simulink model "Improved_version_succesful2"  (Simulink 7.3)
settings: Solver=ode45  StartTime=0.0  StopTime=.25  RelTol=1e-3
values from neighbouring files (symbols this model uses):
  y = 0.01    [objectivefcn.m]
undefined symbols (not defined in the file or in its folder): x
libraries: powerlib x176, powerlib_extras x120
(part 1 of 3)
settings Model: Creator=me  LastModifiedBy=me

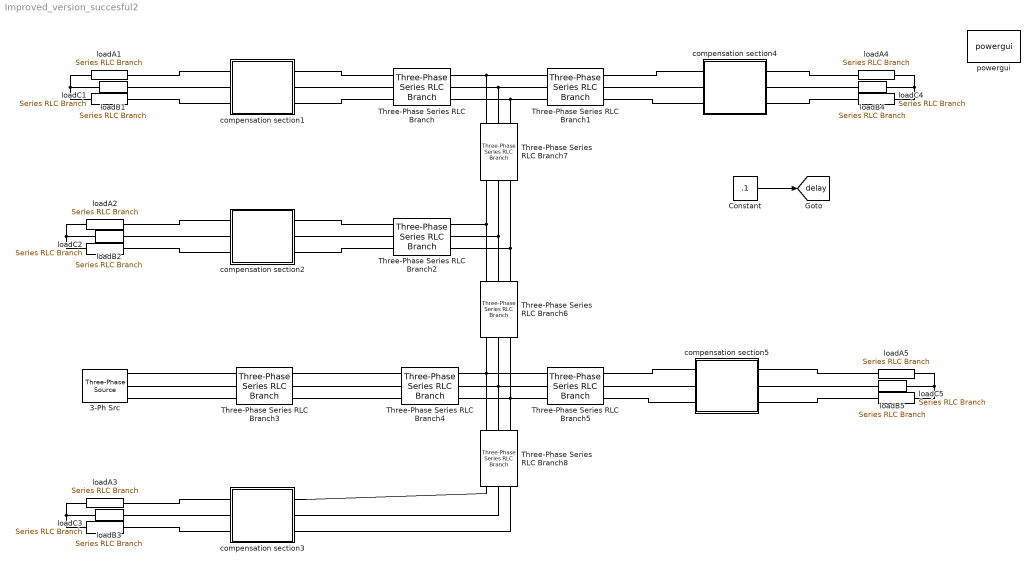
== system Improved_version_succesful2 ==
  3-Ph Src : powerlib/Electrical Sources/Three-Phase Source  DialogController=POWERSYS.PowerSysDialog  SystemSampleTime=-1  Voltage=380  PhaseAngle=0  Frequency=50  InternalConnection=Yn  SpecifyImpedance=on  Resistance=0.8929  Inductance=16.58e-3  ShortCircuitLevel=100e6  BaseVoltage=380  XRratio=7
  Constant : Constant  Value=.1  OutDataType=fixdt(1, 16)  OutScaling=2^0
  Three-Phase Series RLC Branch{,1..8} (9 alike) : powerlib/Elements/Three-Phase Series RLC Branch  DialogController=POWERSYS.PowerSysDialog  PhysicalDomain=powersysdomain  SubClassName=unknown  LeftPortType=p1  RightPortType=p1  LConnTagsString=A|B|C  RConnTagsString=A|B|C  BranchType=RL  Resistance=1  Inductance=1e-3  Capacitance=1e-6  Measurements=None
  compensation section1 : Subsystem
  compensation section2 : Subsystem
  compensation section3 : Subsystem
  compensation section4 : Subsystem
  compensation section5 : Subsystem
  loadA1 : powerlib/Elements/Series RLC Branch  DialogController=POWERSYS.PowerSysDialog  PhysicalDomain=powersysdomain  SubClassName=unknown  LeftPortType=p1  RightPortType=p1  LConnTagsString=__new0  RConnTagsString=__new0  BranchType=Open circuit  Resistance=10  Inductance=30/(100*pi)  SetiL0=off  InitialCurrent=0  Capacitance=1/(100*pi)  Setx0=off  InitialVoltage=0  Measurements=None
  loadA2 : powerlib/Elements/Series RLC Branch  DialogController=POWERSYS.PowerSysDialog  PhysicalDomain=powersysdomain  SubClassName=unknown  LeftPortType=p1  RightPortType=p1  LConnTagsString=__new0  RConnTagsString=__new0  BranchType=RL  Resistance=25  Inductance=30/(100*pi)  SetiL0=off  InitialCurrent=0  Capacitance=1/(100*pi)  Setx0=off  InitialVoltage=0  Measurements=None
  loadA3 : powerlib/Elements/Series RLC Branch  DialogController=POWERSYS.PowerSysDialog  PhysicalDomain=powersysdomain  SubClassName=unknown  LeftPortType=p1  RightPortType=p1  LConnTagsString=__new0  RConnTagsString=__new0  BranchType=R  Resistance=42  Inductance=30/(100*pi)  SetiL0=off  InitialCurrent=0  Capacitance=1/(100*pi)  Setx0=off  InitialVoltage=0  Measurements=None
  loadA4 : powerlib/Elements/Series RLC Branch  DialogController=POWERSYS.PowerSysDialog  PhysicalDomain=powersysdomain  SubClassName=unknown  LeftPortType=p1  RightPortType=p1  LConnTagsString=__new0  RConnTagsString=__new0  BranchType=RL  Resistance=10  Inductance=3/(100*pi)  SetiL0=off  InitialCurrent=0  Capacitance=1/(100*pi)  Setx0=off  InitialVoltage=0  Measurements=None
  loadA5 : powerlib/Elements/Series RLC Branch  DialogController=POWERSYS.PowerSysDialog  PhysicalDomain=powersysdomain  SubClassName=unknown  LeftPortType=p1  RightPortType=p1  LConnTagsString=__new0  RConnTagsString=__new0  BranchType=RL  Resistance=27  Inductance=35/(100*pi)  SetiL0=off  InitialCurrent=0  Capacitance=1/(100*pi)  Setx0=off  InitialVoltage=0  Measurements=None
  loadB1 : powerlib/Elements/Series RLC Branch  DialogController=POWERSYS.PowerSysDialog  PhysicalDomain=powersysdomain  SubClassName=unknown  LeftPortType=p1  RightPortType=p1  LConnTagsString=__new0  RConnTagsString=__new0  BranchType=RC  Resistance=23  Inductance=50/(100*pi)  SetiL0=off  InitialCurrent=0  Capacitance=1/(1200*pi)  Setx0=off  InitialVoltage=0  Measurements=None
  loadB2 : powerlib/Elements/Series RLC Branch  DialogController=POWERSYS.PowerSysDialog  PhysicalDomain=powersysdomain  SubClassName=unknown  LeftPortType=p1  RightPortType=p1  LConnTagsString=__new0  RConnTagsString=__new0  BranchType=R  Resistance=31  Inductance=50/(100*pi)  SetiL0=off  InitialCurrent=0  Capacitance=1/(1200*pi)  Setx0=off  InitialVoltage=0  Measurements=None
  loadB3 : powerlib/Elements/Series RLC Branch  DialogController=POWERSYS.PowerSysDialog  PhysicalDomain=powersysdomain  SubClassName=unknown  LeftPortType=p1  RightPortType=p1  LConnTagsString=__new0  RConnTagsString=__new0  BranchType=C  Resistance=23  Inductance=50/(100*pi)  SetiL0=off  InitialCurrent=0  Capacitance=1/(1200*pi)  Setx0=off  InitialVoltage=0  Measurements=None
  loadB4 : powerlib/Elements/Series RLC Branch  DialogController=POWERSYS.PowerSysDialog  PhysicalDomain=powersysdomain  SubClassName=unknown  LeftPortType=p1  RightPortType=p1  LConnTagsString=__new0  RConnTagsString=__new0  BranchType=LC  Resistance=23  Inductance=12/(100*pi)  SetiL0=off  InitialCurrent=0  Capacitance=1/(2300*pi)  Setx0=off  InitialVoltage=0  Measurements=None
  loadB5 : powerlib/Elements/Series RLC Branch  DialogController=POWERSYS.PowerSysDialog  PhysicalDomain=powersysdomain  SubClassName=unknown  LeftPortType=p1  RightPortType=p1  LConnTagsString=__new0  RConnTagsString=__new0  BranchType=Open circuit  Resistance=23  Inductance=50/(100*pi)  SetiL0=off  InitialCurrent=0  Capacitance=1/(1200*pi)  Setx0=off  InitialVoltage=0  Measurements=None
  loadC1 : powerlib/Elements/Series RLC Branch  DialogController=POWERSYS.PowerSysDialog  PhysicalDomain=powersysdomain  SubClassName=unknown  LeftPortType=p1  RightPortType=p1  LConnTagsString=__new0  RConnTagsString=__new0  BranchType=RL  Resistance=14  Inductance=29/(100*pi)  SetiL0=off  InitialCurrent=0  Capacitance=1.0  Setx0=off  InitialVoltage=0  Measurements=None
  loadC2 : powerlib/Elements/Series RLC Branch  DialogController=POWERSYS.PowerSysDialog  PhysicalDomain=powersysdomain  SubClassName=unknown  LeftPortType=p1  RightPortType=p1  LConnTagsString=__new0  RConnTagsString=__new0  BranchType=RC  Resistance=14  Inductance=29/(100*pi)  SetiL0=off  InitialCurrent=0  Capacitance=1/(1000*pi)  Setx0=off  InitialVoltage=0  Measurements=None
  loadC3 : powerlib/Elements/Series RLC Branch  DialogController=POWERSYS.PowerSysDialog  PhysicalDomain=powersysdomain  SubClassName=unknown  LeftPortType=p1  RightPortType=p1  LConnTagsString=__new0  RConnTagsString=__new0  BranchType=RL  Resistance=14  Inductance=38/(100*pi)  SetiL0=off  InitialCurrent=0  Capacitance=1.0  Setx0=off  InitialVoltage=0  Measurements=None
  loadC4 : powerlib/Elements/Series RLC Branch  DialogController=POWERSYS.PowerSysDialog  PhysicalDomain=powersysdomain  SubClassName=unknown  LeftPortType=p1  RightPortType=p1  LConnTagsString=__new0  RConnTagsString=__new0  BranchType=Open circuit  Resistance=14  Inductance=29/(100*pi)  SetiL0=off  InitialCurrent=0  Capacitance=1  Setx0=off  InitialVoltage=0  Measurements=None
  loadC5 : powerlib/Elements/Series RLC Branch  DialogController=POWERSYS.PowerSysDialog  PhysicalDomain=powersysdomain  SubClassName=unknown  LeftPortType=p1  RightPortType=p1  LConnTagsString=__new0  RConnTagsString=__new0  BranchType=RC  Resistance=24  Inductance=29/(100*pi)  SetiL0=off  InitialCurrent=0  Capacitance=1/(100*pi)  Setx0=off  InitialVoltage=0  Measurements=None
  powergui : powerlib/powergui  Priority=1  SystemSampleTime=-1  SimulationMode=Continuous  SampleTime=50e-6  frequency=60  SPID=off  DisableSnubberDevices=off  DisableRonSwitches=off  DisableVfSwitches=off  SwTol=0  Interpol=off  frequencyindice=50  echomessages=off  HookPort=off  DisplayEquations=off  FunctionMessages=off  EnableUseOfTLC=off  x0status=blocks  RestoreLinks=warning  Frange=[0:2:500]  Ylog=off  Xlog=on  ShowGrid=off  save=off  variable=ZData  ZoomFFT=on  StartTime=0.0  cycles=1  DisplayStyle=1  fundamental=60  FreqAxis=off  MaxFrequency=1000  frequencyindicesteady=1  RmsSteady=1  display=off  Ts=0  methode=off
  tag scope: delay=global
  wires:
  Constant/1 -> [delay]
  connections:
  loadA1/RConn1 -- loadC1/RConn1 -- loadB1/RConn1
  loadB2/RConn1 -- loadA2/RConn1 -- loadC2/RConn1
  loadB3/RConn1 -- loadA3/RConn1 -- loadC3/RConn1
  loadA4/LConn1 -- loadC4/LConn1 -- loadB4/LConn1
  loadB5/LConn1 -- loadA5/LConn1 -- loadC5/LConn1
  3-Ph Src/RConn3 -- Three-Phase Series RLC Branch3/LConn3
  3-Ph Src/RConn2 -- Three-Phase Series RLC Branch3/LConn2
  3-Ph Src/RConn1 -- Three-Phase Series RLC Branch3/LConn1
  Three-Phase Series RLC Branch3/RConn1 -- Three-Phase Series RLC Branch4/LConn1
  Three-Phase Series RLC Branch3/RConn2 -- Three-Phase Series RLC Branch4/LConn2
  Three-Phase Series RLC Branch3/RConn3 -- Three-Phase Series RLC Branch4/LConn3
  Three-Phase Series RLC Branch8/LConn1 -- Three-Phase Series RLC Branch4/RConn1 -- Three-Phase Series RLC Branch5/LConn1 -- Three-Phase Series RLC Branch6/RConn1
  Three-Phase Series RLC Branch8/LConn2 -- Three-Phase Series RLC Branch4/RConn2 -- Three-Phase Series RLC Branch5/LConn2 -- Three-Phase Series RLC Branch6/RConn2
  Three-Phase Series RLC Branch8/LConn3 -- Three-Phase Series RLC Branch4/RConn3 -- Three-Phase Series RLC Branch5/LConn3 -- Three-Phase Series RLC Branch6/RConn3
  Three-Phase Series RLC Branch7/RConn1 -- Three-Phase Series RLC Branch2/RConn1 -- Three-Phase Series RLC Branch6/LConn1
  Three-Phase Series RLC Branch7/RConn2 -- Three-Phase Series RLC Branch2/RConn2 -- Three-Phase Series RLC Branch6/LConn2
  Three-Phase Series RLC Branch7/RConn3 -- Three-Phase Series RLC Branch2/RConn3 -- Three-Phase Series RLC Branch6/LConn3
  Three-Phase Series RLC Branch7/LConn1 -- Three-Phase Series RLC Branch/RConn1 -- Three-Phase Series RLC Branch1/LConn1
  Three-Phase Series RLC Branch7/LConn2 -- Three-Phase Series RLC Branch/RConn2 -- Three-Phase Series RLC Branch1/LConn2
  Three-Phase Series RLC Branch7/LConn3 -- Three-Phase Series RLC Branch/RConn3 -- Three-Phase Series RLC Branch1/LConn3
  compensation section1/LConn1 -- Three-Phase Series RLC Branch/LConn1
  compensation section1/LConn2 -- Three-Phase Series RLC Branch/LConn2
  compensation section1/LConn3 -- Three-Phase Series RLC Branch/LConn3
  compensation section1/RConn1 -- loadA1/LConn1
  compensation section1/RConn2 -- loadB1/LConn1
  loadC1/LConn1 -- compensation section1/RConn3
  compensation section2/LConn2 -- Three-Phase Series RLC Branch2/LConn2
  compensation section2/LConn3 -- Three-Phase Series RLC Branch2/LConn3
  compensation section2/RConn1 -- loadA2/LConn1
  loadB2/LConn1 -- compensation section2/RConn2
  compensation section2/RConn3 -- loadC2/LConn1
  compensation section3/RConn1 -- loadA3/LConn1
  compensation section3/RConn2 -- loadB3/LConn1
  compensation section3/RConn3 -- loadC3/LConn1
  compensation section3/LConn1 -- Three-Phase Series RLC Branch8/RConn1
  Three-Phase Series RLC Branch8/RConn2 -- compensation section3/LConn2
  Three-Phase Series RLC Branch8/RConn3 -- compensation section3/LConn3
  Three-Phase Series RLC Branch2/LConn1 -- compensation section2/LConn1
  compensation section4/LConn1 -- Three-Phase Series RLC Branch1/RConn1
  compensation section4/LConn2 -- Three-Phase Series RLC Branch1/RConn2
  Three-Phase Series RLC Branch1/RConn3 -- compensation section4/LConn3
  compensation section4/RConn1 -- loadA4/RConn1
  compensation section4/RConn2 -- loadB4/RConn1
  compensation section4/RConn3 -- loadC4/RConn1
  compensation section5/LConn1 -- Three-Phase Series RLC Branch5/RConn1
  Three-Phase Series RLC Branch5/RConn2 -- compensation section5/LConn2
  Three-Phase Series RLC Branch5/RConn3 -- compensation section5/LConn3
  compensation section5/RConn1 -- loadA5/RConn1
  compensation section5/RConn2 -- loadB5/RConn1
  compensation section5/RConn3 -- loadC5/RConn1

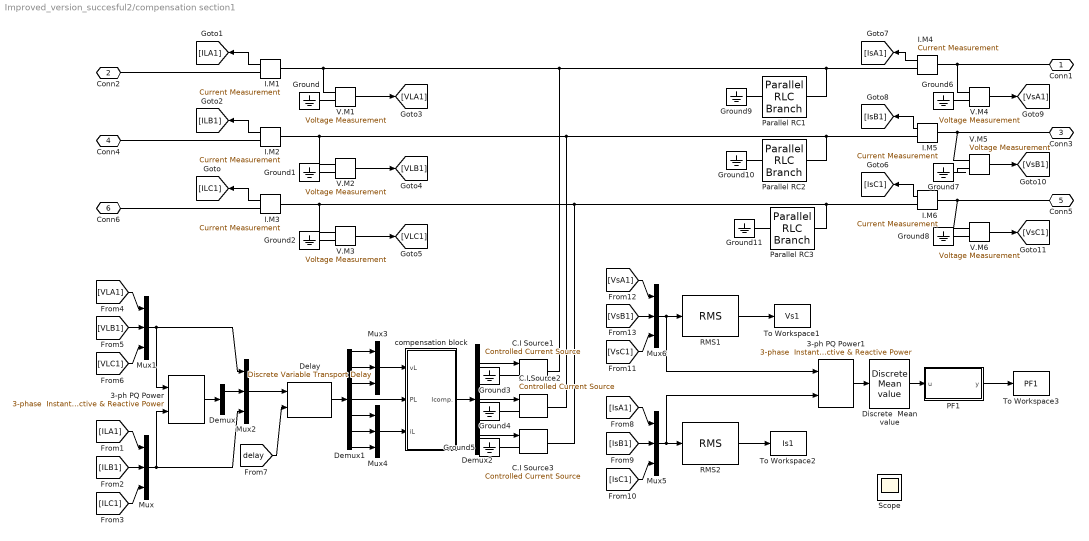
== system Improved_version_succesful2/compensation section1 ==
  3-ph PQ Power : powerlib_extras/Measurements/3-phase  Instantaneous  Active & Reactive Power  DialogController=POWERSYS.PowerSysDialog  SystemSampleTime=-1
  3-ph PQ Power1 : powerlib_extras/Measurements/3-phase  Instantaneous  Active & Reactive Power  DialogController=POWERSYS.PowerSysDialog  SystemSampleTime=-1
  C.I Source1 : powerlib/Electrical Sources/Controlled Current Source  DialogController=POWERSYS.PowerSysDialog  SystemSampleTime=-1  Initialize=on  Source_Type=AC  Amplitude=0  Phase=0  Frequency=0  Measurements=None
  C.I Source2 : powerlib/Electrical Sources/Controlled Current Source  DialogController=POWERSYS.PowerSysDialog  SystemSampleTime=-1  Initialize=on  Source_Type=AC  Amplitude=0  Phase=0  Frequency=0  Measurements=None
  C.I Source3 : powerlib/Electrical Sources/Controlled Current Source  DialogController=POWERSYS.PowerSysDialog  SystemSampleTime=-1  Initialize=on  Source_Type=AC  Amplitude=0  Phase=0  Frequency=0  Measurements=None
  Delay : powerlib_extras/Discrete  Control Blocks/Discrete Variable Transport Delay  DialogController=POWERSYS.PowerSysDialog  SystemSampleTime=-1  MaxDelay=1/40  InitialValue=0  Ts=50e-6
  Demux : Demux  Outputs=2
  Demux1 : Demux  Outputs=7
  Demux2 : Demux  Outputs=3
  Discrete  Mean value : powerlib_extras/Discrete Measurements/Discrete  Mean value  DialogController=POWERSYS.PowerSysDialog  SystemSampleTime=-1  Freq=50  Vinit=0  Ts=50e-6
  Ground{,1..11} (12 alike) : powerlib/Elements/Ground  DialogController=POWERSYS.PowerSysDialog  PhysicalDomain=powersysdomain  SubClassName=unknown  LeftPortType=p1  RightPortType=p1  LConnTagsString=a
  I.M{1..6} (6 alike) : powerlib/Measurements/Current Measurement  DialogController=POWERSYS.PowerSysDialog  SystemSampleTime=-1  PhasorSimulation=off  OutputType=Complex  PSBequivalent=0
  Mux{,1..6} (7 alike) : Mux  Inputs=3
  PF1 : Stateflow chart
  Parallel RC1 : powerlib/Elements/Parallel RLC Branch  DialogController=POWERSYS.PowerSysDialog  PhysicalDomain=powersysdomain  SubClassName=unknown  LeftPortType=p1  RightPortType=p1  LConnTagsString=a  RConnTagsString=__new0  BranchType=RC  Resistance=100  Inductance=1e-3  SetiL0=off  InitialCurrent=0  Capacitance=1/(10000*pi)  Setx0=off  InitialVoltage=0  Measurements=None
  Parallel RC2 : powerlib/Elements/Parallel RLC Branch  DialogController=POWERSYS.PowerSysDialog  PhysicalDomain=powersysdomain  SubClassName=unknown  LeftPortType=p1  RightPortType=p1  LConnTagsString=a  RConnTagsString=__new0  BranchType=RC  Resistance=100  Inductance=1e-3  SetiL0=off  InitialCurrent=0  Capacitance=1/(10000*pi)  Setx0=off  InitialVoltage=0  Measurements=None
  Parallel RC3 : powerlib/Elements/Parallel RLC Branch  DialogController=POWERSYS.PowerSysDialog  PhysicalDomain=powersysdomain  SubClassName=unknown  LeftPortType=p1  RightPortType=p1  LConnTagsString=a  RConnTagsString=__new0  BranchType=RC  Resistance=100  Inductance=1e-3  SetiL0=off  InitialCurrent=0  Capacitance=1/(10000*pi)  Setx0=off  InitialVoltage=0  Measurements=None
  RMS1 : powerlib_extras/Measurements/RMS  DialogController=POWERSYS.PowerSysDialog  SystemSampleTime=-1  f1=50
  RMS2 : powerlib_extras/Measurements/RMS  DialogController=POWERSYS.PowerSysDialog  SystemSampleTime=-1  f1=50
  Scope : Scope
      settings: YMin=2  YMax=6  SaveName=ScopeData2
  To Workspace1 : ToWorkspace  VariableName=Vs1  SampleTime=y  SaveFormat=Array
  To Workspace2 : ToWorkspace  VariableName=Is1  SampleTime=y  SaveFormat=Array
  To Workspace3 : ToWorkspace  VariableName=PF1  SampleTime=y  SaveFormat=Array
  V.M{1..6} (6 alike) : powerlib/Measurements/Voltage Measurement  DialogController=POWERSYS.PowerSysDialog  SystemSampleTime=-1  PhasorSimulation=off  OutputType=Complex  PSBequivalent=0
  compensation block : Subsystem
  Conn1 : PMIOPort  Port=1  Side=Left
  Conn2 : PMIOPort  Port=2  Side=Right
  Conn3 : PMIOPort  Port=3  Side=Left
  Conn4 : PMIOPort  Port=4  Side=Right
  Conn5 : PMIOPort  Port=5  Side=Left
  Conn6 : PMIOPort  Port=6  Side=Right
  wires:
  I.M1/1 -> [ILA1]
  I.M2/1 -> [ILB1]
  V.M1/1 -> [VLA1]
  V.M2/1 -> [VLB1]
  V.M3/1 -> [VLC1]
  [ILB1] -> Mux/2
  [ILA1] -> Mux/1
  [ILC1] -> Mux/3
  [VLB1] -> Mux1/2
  [VLA1] -> Mux1/1
  [VLC1] -> Mux1/3
  Mux1/1 -> Mux2/1, 3-ph PQ Power/1
  Mux/1 -> Mux2/3, 3-ph PQ Power/2
  3-ph PQ Power/1 -> Demux/1
  Demux/1 -> Mux2/2
  Mux2/1 -> Delay/1
  [delay] -> Delay/2
  Delay/1 -> Demux1/1
  Demux1/6 -> Mux4/2
  Demux1/5 -> Mux4/1
  Demux1/7 -> Mux4/3
  Demux1/1 -> Mux3/1
  Demux1/2 -> Mux3/2
  Demux1/3 -> Mux3/3
  Mux3/1 -> compensation block/1(vL)
  Demux1/4 -> compensation block/2(PL)
  Mux4/1 -> compensation block/3(iL)
  compensation block/1(Icomp.) -> Demux2/1
  Demux2/1 -> C.I Source1/1
  Demux2/2 -> C.I Source2/1
  Demux2/3 -> C.I Source3/1
  I.M3/1 -> [ILC1]
  I.M5/1 -> [IsB1]
  V.M4/1 -> [VsA1]
  V.M5/1 -> [VsB1]
  V.M6/1 -> [VsC1]
  I.M6/1 -> [IsC1]
  I.M4/1 -> [IsA1]
  [VsB1] -> Mux6/2
  [VsA1] -> Mux6/1
  [VsC1] -> Mux6/3
  Mux6/1 -> RMS1/1, 3-ph PQ Power1/1
  RMS1/1 -> To Workspace1/1
  [IsB1] -> Mux5/2
  [IsA1] -> Mux5/1
  [IsC1] -> Mux5/3
  Mux5/1 -> RMS2/1, 3-ph PQ Power1/2
  RMS2/1 -> To Workspace2/1
  3-ph PQ Power1/1 -> Discrete  Mean value/1
  Discrete  Mean value/1 -> PF1/1(u)
  PF1/1(y) -> To Workspace3/1
  connections:
  I.M1/LConn1 -- V.M1/LConn1 -- I.M4/RConn1 -- Parallel RC1/RConn1 -- C.I Source1/RConn1
  Conn2/RConn1 -- I.M1/RConn1
  I.M2/LConn1 -- V.M2/LConn1 -- I.M5/RConn1 -- Parallel RC2/RConn1 -- C.I Source2/RConn1
  Conn4/RConn1 -- I.M2/RConn1
  I.M3/LConn1 -- V.M3/LConn1 -- I.M6/RConn1 -- Parallel RC3/RConn1 -- C.I Source3/RConn1
  Ground/LConn1 -- V.M1/LConn2
  Ground1/LConn1 -- V.M2/LConn2
  Ground2/LConn1 -- V.M3/LConn2
  Ground5/LConn1 -- C.I Source3/LConn1
  Ground4/LConn1 -- C.I Source2/LConn1
  Ground3/LConn1 -- C.I Source1/LConn1
  Conn6/RConn1 -- I.M3/RConn1
  Conn1/RConn1 -- V.M4/LConn1 -- I.M4/LConn1
  V.M5/LConn1 -- I.M5/LConn1 -- Conn3/RConn1
  V.M6/LConn1 -- I.M6/LConn1 -- Conn5/RConn1
  Ground6/LConn1 -- V.M4/LConn2
  Ground7/LConn1 -- V.M5/LConn2
  Ground8/LConn1 -- V.M6/LConn2
  Parallel RC3/LConn1 -- Ground11/LConn1
  Parallel RC2/LConn1 -- Ground10/LConn1
  Parallel RC1/LConn1 -- Ground9/LConn1

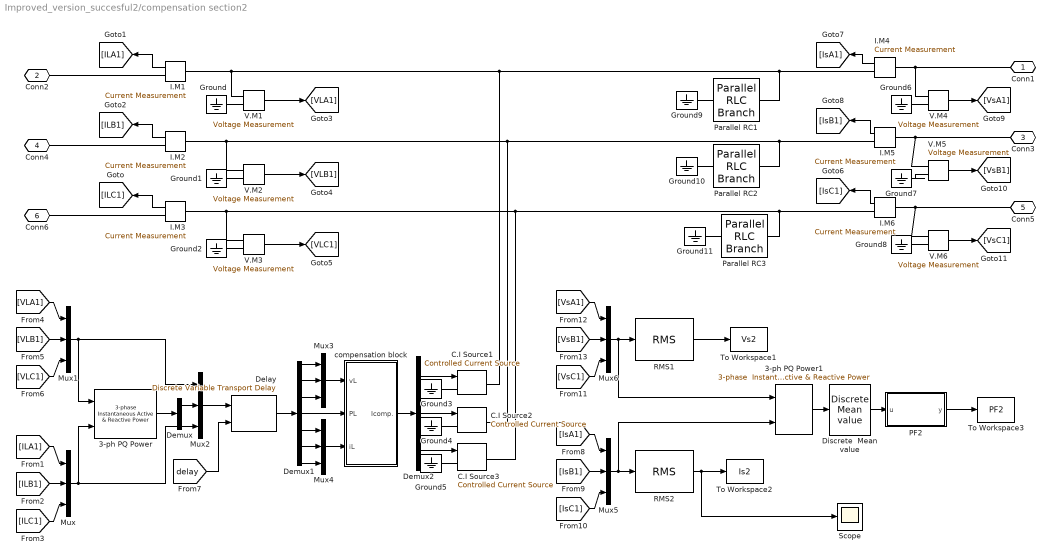
== system Improved_version_succesful2/compensation section2 ==
  3-ph PQ Power : powerlib_extras/Measurements/3-phase  Instantaneous  Active & Reactive Power  DialogController=POWERSYS.PowerSysDialog  SystemSampleTime=-1
  3-ph PQ Power1 : powerlib_extras/Measurements/3-phase  Instantaneous  Active & Reactive Power  DialogController=POWERSYS.PowerSysDialog  SystemSampleTime=-1
  C.I Source1 : powerlib/Electrical Sources/Controlled Current Source  DialogController=POWERSYS.PowerSysDialog  SystemSampleTime=-1  Initialize=on  Source_Type=AC  Amplitude=0  Phase=0  Frequency=0  Measurements=None
  C.I Source2 : powerlib/Electrical Sources/Controlled Current Source  DialogController=POWERSYS.PowerSysDialog  SystemSampleTime=-1  Initialize=on  Source_Type=AC  Amplitude=0  Phase=0  Frequency=0  Measurements=None
  C.I Source3 : powerlib/Electrical Sources/Controlled Current Source  DialogController=POWERSYS.PowerSysDialog  SystemSampleTime=-1  Initialize=on  Source_Type=AC  Amplitude=0  Phase=0  Frequency=0  Measurements=None
  Delay : powerlib_extras/Discrete  Control Blocks/Discrete Variable Transport Delay  DialogController=POWERSYS.PowerSysDialog  SystemSampleTime=-1  MaxDelay=1/40  InitialValue=0  Ts=50e-6
  Demux : Demux  Outputs=2
  Demux1 : Demux  Outputs=7
  Demux2 : Demux  Outputs=3
  Discrete  Mean value : powerlib_extras/Discrete Measurements/Discrete  Mean value  DialogController=POWERSYS.PowerSysDialog  SystemSampleTime=-1  Freq=50  Vinit=0  Ts=50e-6
  Ground{,1..11} (12 alike) : powerlib/Elements/Ground  DialogController=POWERSYS.PowerSysDialog  PhysicalDomain=powersysdomain  SubClassName=unknown  LeftPortType=p1  RightPortType=p1  LConnTagsString=a
  I.M{1..6} (6 alike) : powerlib/Measurements/Current Measurement  DialogController=POWERSYS.PowerSysDialog  SystemSampleTime=-1  PhasorSimulation=off  OutputType=Complex  PSBequivalent=0
  Mux{,1..6} (7 alike) : Mux  Inputs=3
  PF2 : Stateflow chart
  Parallel RC1 : powerlib/Elements/Parallel RLC Branch  DialogController=POWERSYS.PowerSysDialog  PhysicalDomain=powersysdomain  SubClassName=unknown  LeftPortType=p1  RightPortType=p1  LConnTagsString=a  RConnTagsString=__new0  BranchType=RC  Resistance=100  Inductance=1e-3  SetiL0=off  InitialCurrent=0  Capacitance=1/(10000*pi)  Setx0=off  InitialVoltage=0  Measurements=None
  Parallel RC2 : powerlib/Elements/Parallel RLC Branch  DialogController=POWERSYS.PowerSysDialog  PhysicalDomain=powersysdomain  SubClassName=unknown  LeftPortType=p1  RightPortType=p1  LConnTagsString=a  RConnTagsString=__new0  BranchType=RC  Resistance=100  Inductance=1e-3  SetiL0=off  InitialCurrent=0  Capacitance=1/(10000*pi)  Setx0=off  InitialVoltage=0  Measurements=None
  Parallel RC3 : powerlib/Elements/Parallel RLC Branch  DialogController=POWERSYS.PowerSysDialog  PhysicalDomain=powersysdomain  SubClassName=unknown  LeftPortType=p1  RightPortType=p1  LConnTagsString=a  RConnTagsString=__new0  BranchType=RC  Resistance=100  Inductance=1e-3  SetiL0=off  InitialCurrent=0  Capacitance=1/(10000*pi)  Setx0=off  InitialVoltage=0  Measurements=None
  RMS1 : powerlib_extras/Measurements/RMS  DialogController=POWERSYS.PowerSysDialog  SystemSampleTime=-1  f1=50
  RMS2 : powerlib_extras/Measurements/RMS  DialogController=POWERSYS.PowerSysDialog  SystemSampleTime=-1  f1=50
  Scope : Scope
      settings: YMin=4  YMax=10  SaveName=ScopeData3
  To Workspace1 : ToWorkspace  VariableName=Vs2  SampleTime=y  SaveFormat=Array
  To Workspace2 : ToWorkspace  VariableName=Is2  SampleTime=y  SaveFormat=Array
  To Workspace3 : ToWorkspace  VariableName=PF2  SampleTime=y  SaveFormat=Array
  V.M{1..6} (6 alike) : powerlib/Measurements/Voltage Measurement  DialogController=POWERSYS.PowerSysDialog  SystemSampleTime=-1  PhasorSimulation=off  OutputType=Complex  PSBequivalent=0
  compensation block : Subsystem
  Conn1 : PMIOPort  Port=1  Side=Left
  Conn2 : PMIOPort  Port=2  Side=Right
  Conn3 : PMIOPort  Port=3  Side=Left
  Conn4 : PMIOPort  Port=4  Side=Right
  Conn5 : PMIOPort  Port=5  Side=Left
  Conn6 : PMIOPort  Port=6  Side=Right
  wires:
  I.M4/1 -> [IsA1]
  I.M6/1 -> [IsC1]
  V.M6/1 -> [VsC1]
  V.M5/1 -> [VsB1]
  V.M4/1 -> [VsA1]
  I.M5/1 -> [IsB1]
  I.M3/1 -> [ILC1]
  Demux2/3 -> C.I Source3/1
  Demux2/2 -> C.I Source2/1
  Demux2/1 -> C.I Source1/1
  compensation block/1(Icomp.) -> Demux2/1
  Mux4/1 -> compensation block/3(iL)
  Demux1/4 -> compensation block/2(PL)
  Mux3/1 -> compensation block/1(vL)
  Demux1/3 -> Mux3/3
  Demux1/2 -> Mux3/2
  Demux1/1 -> Mux3/1
  Demux1/7 -> Mux4/3
  Demux1/5 -> Mux4/1
  Demux1/6 -> Mux4/2
  Delay/1 -> Demux1/1
  [delay] -> Delay/2
  Mux2/1 -> Delay/1
  Demux/1 -> Mux2/2
  3-ph PQ Power/1 -> Demux/1
  Mux/1 -> Mux2/3, 3-ph PQ Power/2
  Mux1/1 -> Mux2/1, 3-ph PQ Power/1
  [VLC1] -> Mux1/3
  [VLA1] -> Mux1/1
  [VLB1] -> Mux1/2
  [ILC1] -> Mux/3
  [ILA1] -> Mux/1
  [ILB1] -> Mux/2
  V.M3/1 -> [VLC1]
  V.M2/1 -> [VLB1]
  V.M1/1 -> [VLA1]
  I.M2/1 -> [ILB1]
  I.M1/1 -> [ILA1]
  [VsB1] -> Mux6/2
  [VsA1] -> Mux6/1
  [VsC1] -> Mux6/3
  Mux6/1 -> RMS1/1, 3-ph PQ Power1/1
  RMS1/1 -> To Workspace1/1
  [IsB1] -> Mux5/2
  [IsA1] -> Mux5/1
  [IsC1] -> Mux5/3
  Mux5/1 -> RMS2/1, 3-ph PQ Power1/2
  RMS2/1 -> To Workspace2/1, Scope/1
  3-ph PQ Power1/1 -> Discrete  Mean value/1
  Discrete  Mean value/1 -> PF2/1(u)
  PF2/1(y) -> To Workspace3/1
  connections:
  Parallel RC1/LConn1 -- Ground9/LConn1
  Parallel RC2/LConn1 -- Ground10/LConn1
  Parallel RC3/LConn1 -- Ground11/LConn1
  Ground8/LConn1 -- V.M6/LConn2
  Ground7/LConn1 -- V.M5/LConn2
  Ground6/LConn1 -- V.M4/LConn2
  Conn5/RConn1 -- I.M6/LConn1 -- V.M6/LConn1
  Conn3/RConn1 -- I.M5/LConn1 -- V.M5/LConn1
  I.M4/LConn1 -- V.M4/LConn1 -- Conn1/RConn1
  Conn6/RConn1 -- I.M3/RConn1
  Ground3/LConn1 -- C.I Source1/LConn1
  Ground4/LConn1 -- C.I Source2/LConn1
  Ground5/LConn1 -- C.I Source3/LConn1
  Ground2/LConn1 -- V.M3/LConn2
  Ground1/LConn1 -- V.M2/LConn2
  Ground/LConn1 -- V.M1/LConn2
  V.M3/LConn1 -- I.M3/LConn1 -- Parallel RC3/RConn1 -- I.M6/RConn1 -- C.I Source3/RConn1
  Conn4/RConn1 -- I.M2/RConn1
  V.M2/LConn1 -- I.M2/LConn1 -- Parallel RC2/RConn1 -- I.M5/RConn1 -- C.I Source2/RConn1
  Conn2/RConn1 -- I.M1/RConn1
  V.M1/LConn1 -- I.M1/LConn1 -- Parallel RC1/RConn1 -- I.M4/RConn1 -- C.I Source1/RConn1

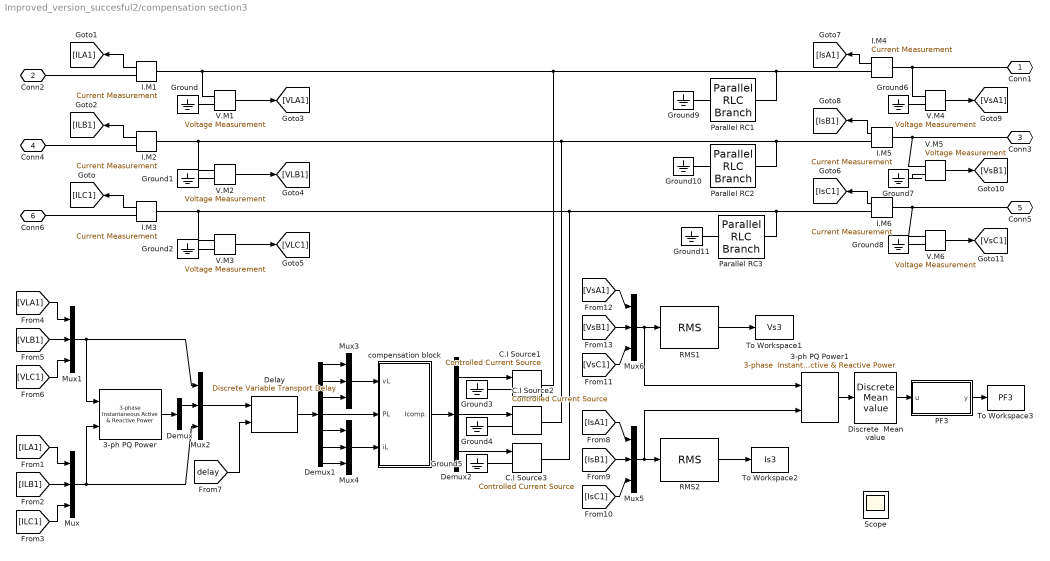
== system Improved_version_succesful2/compensation section3 ==
  3-ph PQ Power : powerlib_extras/Measurements/3-phase  Instantaneous  Active & Reactive Power  DialogController=POWERSYS.PowerSysDialog  SystemSampleTime=-1
  3-ph PQ Power1 : powerlib_extras/Measurements/3-phase  Instantaneous  Active & Reactive Power  DialogController=POWERSYS.PowerSysDialog  SystemSampleTime=-1
  C.I Source1 : powerlib/Electrical Sources/Controlled Current Source  DialogController=POWERSYS.PowerSysDialog  SystemSampleTime=-1  Initialize=on  Source_Type=AC  Amplitude=0  Phase=0  Frequency=0  Measurements=None
  C.I Source2 : powerlib/Electrical Sources/Controlled Current Source  DialogController=POWERSYS.PowerSysDialog  SystemSampleTime=-1  Initialize=on  Source_Type=AC  Amplitude=0  Phase=0  Frequency=0  Measurements=None
  C.I Source3 : powerlib/Electrical Sources/Controlled Current Source  DialogController=POWERSYS.PowerSysDialog  SystemSampleTime=-1  Initialize=on  Source_Type=AC  Amplitude=0  Phase=0  Frequency=0  Measurements=None
  Delay : powerlib_extras/Discrete  Control Blocks/Discrete Variable Transport Delay  DialogController=POWERSYS.PowerSysDialog  SystemSampleTime=-1  MaxDelay=1/40  InitialValue=0  Ts=50e-6
  Demux : Demux  Outputs=2
  Demux1 : Demux  Outputs=7
  Demux2 : Demux  Outputs=3
  Discrete  Mean value : powerlib_extras/Discrete Measurements/Discrete  Mean value  DialogController=POWERSYS.PowerSysDialog  SystemSampleTime=-1  Freq=50  Vinit=0  Ts=50e-6
  Ground{,1..11} (12 alike) : powerlib/Elements/Ground  DialogController=POWERSYS.PowerSysDialog  PhysicalDomain=powersysdomain  SubClassName=unknown  LeftPortType=p1  RightPortType=p1  LConnTagsString=a
  I.M{1..6} (6 alike) : powerlib/Measurements/Current Measurement  DialogController=POWERSYS.PowerSysDialog  SystemSampleTime=-1  PhasorSimulation=off  OutputType=Complex  PSBequivalent=0
  Mux{,1..6} (7 alike) : Mux  Inputs=3
  PF3 : Stateflow chart
  Parallel RC1 : powerlib/Elements/Parallel RLC Branch  DialogController=POWERSYS.PowerSysDialog  PhysicalDomain=powersysdomain  SubClassName=unknown  LeftPortType=p1  RightPortType=p1  LConnTagsString=a  RConnTagsString=__new0  BranchType=RC  Resistance=100  Inductance=1e-3  SetiL0=off  InitialCurrent=0  Capacitance=1/(10000*pi)  Setx0=off  InitialVoltage=0  Measurements=None
  Parallel RC2 : powerlib/Elements/Parallel RLC Branch  DialogController=POWERSYS.PowerSysDialog  PhysicalDomain=powersysdomain  SubClassName=unknown  LeftPortType=p1  RightPortType=p1  LConnTagsString=a  RConnTagsString=__new0  BranchType=RC  Resistance=100  Inductance=1e-3  SetiL0=off  InitialCurrent=0  Capacitance=1/(10000*pi)  Setx0=off  InitialVoltage=0  Measurements=None
  Parallel RC3 : powerlib/Elements/Parallel RLC Branch  DialogController=POWERSYS.PowerSysDialog  PhysicalDomain=powersysdomain  SubClassName=unknown  LeftPortType=p1  RightPortType=p1  LConnTagsString=a  RConnTagsString=__new0  BranchType=RC  Resistance=100  Inductance=1e-3  SetiL0=off  InitialCurrent=0  Capacitance=1/(10000*pi)  Setx0=off  InitialVoltage=0  Measurements=None
  RMS1 : powerlib_extras/Measurements/RMS  DialogController=POWERSYS.PowerSysDialog  SystemSampleTime=-1  f1=50
  RMS2 : powerlib_extras/Measurements/RMS  DialogController=POWERSYS.PowerSysDialog  SystemSampleTime=-1  f1=50
  Scope : Scope
      settings: YMin=2  YMax=6  SaveName=ScopeData4
  To Workspace1 : ToWorkspace  VariableName=Vs3  SampleTime=y  SaveFormat=Array
  To Workspace2 : ToWorkspace  VariableName=Is3  SampleTime=y  SaveFormat=Array
  To Workspace3 : ToWorkspace  VariableName=PF3  SampleTime=y  SaveFormat=Array
  V.M{1..6} (6 alike) : powerlib/Measurements/Voltage Measurement  DialogController=POWERSYS.PowerSysDialog  SystemSampleTime=-1  PhasorSimulation=off  OutputType=Complex  PSBequivalent=0
  compensation block : Subsystem
  Conn1 : PMIOPort  Port=1  Side=Left
  Conn2 : PMIOPort  Port=2  Side=Right
  Conn3 : PMIOPort  Port=3  Side=Left
  Conn4 : PMIOPort  Port=4  Side=Right
  Conn5 : PMIOPort  Port=5  Side=Left
  Conn6 : PMIOPort  Port=6  Side=Right
  wires:
  I.M1/1 -> [ILA1]
  I.M2/1 -> [ILB1]
  V.M1/1 -> [VLA1]
  V.M2/1 -> [VLB1]
  V.M3/1 -> [VLC1]
  [ILB1] -> Mux/2
  [ILA1] -> Mux/1
  [ILC1] -> Mux/3
  [VLB1] -> Mux1/2
  [VLA1] -> Mux1/1
  [VLC1] -> Mux1/3
  Mux1/1 -> 3-ph PQ Power/1, Mux2/1
  Mux/1 -> 3-ph PQ Power/2, Mux2/3
  3-ph PQ Power/1 -> Demux/1
  Demux/1 -> Mux2/2
  Mux2/1 -> Delay/1
  [delay] -> Delay/2
  Delay/1 -> Demux1/1
  Demux1/6 -> Mux4/2
  Demux1/5 -> Mux4/1
  Demux1/7 -> Mux4/3
  Demux1/1 -> Mux3/1
  Demux1/2 -> Mux3/2
  Demux1/3 -> Mux3/3
  Mux3/1 -> compensation block/1(vL)
  Demux1/4 -> compensation block/2(PL)
  Mux4/1 -> compensation block/3(iL)
  compensation block/1(Icomp.) -> Demux2/1
  Demux2/1 -> C.I Source1/1
  Demux2/2 -> C.I Source2/1
  Demux2/3 -> C.I Source3/1
  I.M3/1 -> [ILC1]
  I.M5/1 -> [IsB1]
  V.M4/1 -> [VsA1]
  V.M5/1 -> [VsB1]
  V.M6/1 -> [VsC1]
  I.M6/1 -> [IsC1]
  I.M4/1 -> [IsA1]
  [VsB1] -> Mux6/2
  [VsA1] -> Mux6/1
  [VsC1] -> Mux6/3
  Mux6/1 -> RMS1/1, 3-ph PQ Power1/1
  RMS1/1 -> To Workspace1/1
  [IsB1] -> Mux5/2
  [IsA1] -> Mux5/1
  [IsC1] -> Mux5/3
  Mux5/1 -> RMS2/1, 3-ph PQ Power1/2
  RMS2/1 -> To Workspace2/1
  3-ph PQ Power1/1 -> Discrete  Mean value/1
  Discrete  Mean value/1 -> PF3/1(u)
  PF3/1(y) -> To Workspace3/1
  connections:
  I.M1/LConn1 -- V.M1/LConn1 -- I.M4/RConn1 -- Parallel RC1/RConn1 -- C.I Source1/RConn1
  Conn2/RConn1 -- I.M1/RConn1
  I.M2/LConn1 -- V.M2/LConn1 -- I.M5/RConn1 -- Parallel RC2/RConn1 -- C.I Source2/RConn1
  Conn4/RConn1 -- I.M2/RConn1
  I.M3/LConn1 -- V.M3/LConn1 -- I.M6/RConn1 -- Parallel RC3/RConn1 -- C.I Source3/RConn1
  Ground/LConn1 -- V.M1/LConn2
  Ground1/LConn1 -- V.M2/LConn2
  Ground2/LConn1 -- V.M3/LConn2
  Ground5/LConn1 -- C.I Source3/LConn1
  Ground4/LConn1 -- C.I Source2/LConn1
  Ground3/LConn1 -- C.I Source1/LConn1
  Conn6/RConn1 -- I.M3/RConn1
  Conn1/RConn1 -- V.M4/LConn1 -- I.M4/LConn1
  V.M5/LConn1 -- I.M5/LConn1 -- Conn3/RConn1
  V.M6/LConn1 -- I.M6/LConn1 -- Conn5/RConn1
  Ground6/LConn1 -- V.M4/LConn2
  Ground7/LConn1 -- V.M5/LConn2
  Ground8/LConn1 -- V.M6/LConn2
  Parallel RC3/LConn1 -- Ground11/LConn1
  Parallel RC2/LConn1 -- Ground10/LConn1
  Parallel RC1/LConn1 -- Ground9/LConn1

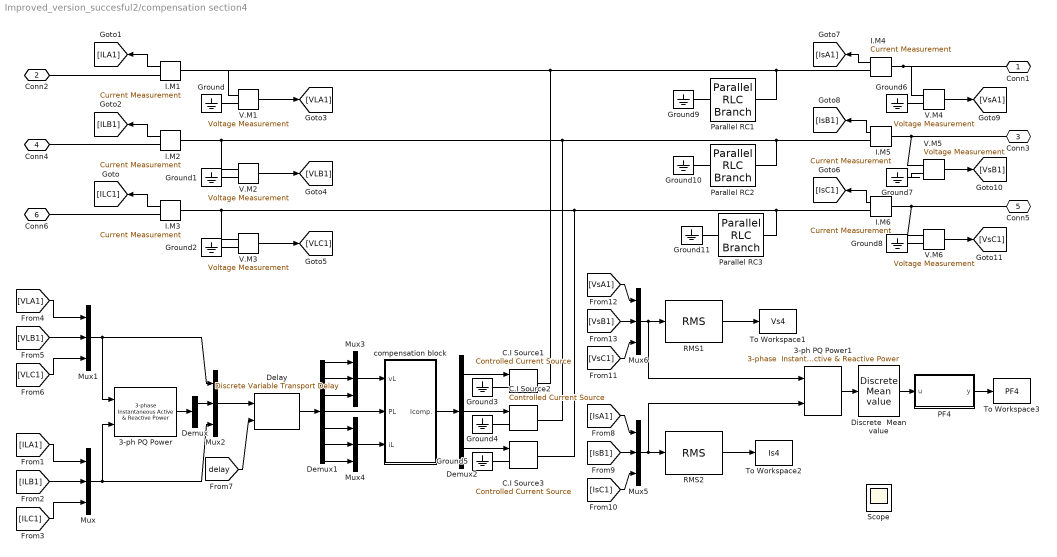
== system Improved_version_succesful2/compensation section4 ==
  3-ph PQ Power : powerlib_extras/Measurements/3-phase  Instantaneous  Active & Reactive Power  DialogController=POWERSYS.PowerSysDialog  SystemSampleTime=-1
  3-ph PQ Power1 : powerlib_extras/Measurements/3-phase  Instantaneous  Active & Reactive Power  DialogController=POWERSYS.PowerSysDialog  SystemSampleTime=-1
  C.I Source1 : powerlib/Electrical Sources/Controlled Current Source  DialogController=POWERSYS.PowerSysDialog  SystemSampleTime=-1  Initialize=on  Source_Type=AC  Amplitude=0  Phase=0  Frequency=0  Measurements=None
  C.I Source2 : powerlib/Electrical Sources/Controlled Current Source  DialogController=POWERSYS.PowerSysDialog  SystemSampleTime=-1  Initialize=on  Source_Type=AC  Amplitude=0  Phase=0  Frequency=0  Measurements=None
  C.I Source3 : powerlib/Electrical Sources/Controlled Current Source  DialogController=POWERSYS.PowerSysDialog  SystemSampleTime=-1  Initialize=on  Source_Type=AC  Amplitude=0  Phase=0  Frequency=0  Measurements=None
  Delay : powerlib_extras/Discrete  Control Blocks/Discrete Variable Transport Delay  DialogController=POWERSYS.PowerSysDialog  SystemSampleTime=-1  MaxDelay=1/40  InitialValue=0  Ts=50e-6
  Demux : Demux  Outputs=2
  Demux1 : Demux  Outputs=7
  Demux2 : Demux  Outputs=3
  Discrete  Mean value : powerlib_extras/Discrete Measurements/Discrete  Mean value  DialogController=POWERSYS.PowerSysDialog  SystemSampleTime=-1  Freq=50  Vinit=0  Ts=50e-6
  Ground{,1..11} (12 alike) : powerlib/Elements/Ground  DialogController=POWERSYS.PowerSysDialog  PhysicalDomain=powersysdomain  SubClassName=unknown  LeftPortType=p1  RightPortType=p1  LConnTagsString=a
  I.M{1..6} (6 alike) : powerlib/Measurements/Current Measurement  DialogController=POWERSYS.PowerSysDialog  SystemSampleTime=-1  PhasorSimulation=off  OutputType=Complex  PSBequivalent=0
  Mux{,1..6} (7 alike) : Mux  Inputs=3
  PF4 : Stateflow chart
  Parallel RC1 : powerlib/Elements/Parallel RLC Branch  DialogController=POWERSYS.PowerSysDialog  PhysicalDomain=powersysdomain  SubClassName=unknown  LeftPortType=p1  RightPortType=p1  LConnTagsString=a  RConnTagsString=__new0  BranchType=RC  Resistance=100  Inductance=1e-3  SetiL0=off  InitialCurrent=0  Capacitance=1/(10000*pi)  Setx0=off  InitialVoltage=0  Measurements=None
  Parallel RC2 : powerlib/Elements/Parallel RLC Branch  DialogController=POWERSYS.PowerSysDialog  PhysicalDomain=powersysdomain  SubClassName=unknown  LeftPortType=p1  RightPortType=p1  LConnTagsString=a  RConnTagsString=__new0  BranchType=RC  Resistance=100  Inductance=1e-3  SetiL0=off  InitialCurrent=0  Capacitance=1/(10000*pi)  Setx0=off  InitialVoltage=0  Measurements=None
  Parallel RC3 : powerlib/Elements/Parallel RLC Branch  DialogController=POWERSYS.PowerSysDialog  PhysicalDomain=powersysdomain  SubClassName=unknown  LeftPortType=p1  RightPortType=p1  LConnTagsString=a  RConnTagsString=__new0  BranchType=RC  Resistance=100  Inductance=1e-3  SetiL0=off  InitialCurrent=0  Capacitance=1/(10000*pi)  Setx0=off  InitialVoltage=0  Measurements=None
  RMS1 : powerlib_extras/Measurements/RMS  DialogController=POWERSYS.PowerSysDialog  SystemSampleTime=-1  f1=50
  RMS2 : powerlib_extras/Measurements/RMS  DialogController=POWERSYS.PowerSysDialog  SystemSampleTime=-1  f1=50
  Scope : Scope
      settings: YMin=2  YMax=6  SaveName=ScopeData5
  To Workspace1 : ToWorkspace  VariableName=Vs4  SampleTime=y  SaveFormat=Array
  To Workspace2 : ToWorkspace  VariableName=Is4  SampleTime=y  SaveFormat=Array
  To Workspace3 : ToWorkspace  VariableName=PF4  SampleTime=y  SaveFormat=Array
  V.M{1..6} (6 alike) : powerlib/Measurements/Voltage Measurement  DialogController=POWERSYS.PowerSysDialog  SystemSampleTime=-1  PhasorSimulation=off  OutputType=Complex  PSBequivalent=0
  compensation block : Subsystem
  Conn1 : PMIOPort  Port=1  Side=Left
  Conn2 : PMIOPort  Port=2  Side=Right
  Conn3 : PMIOPort  Port=3  Side=Left
  Conn4 : PMIOPort  Port=4  Side=Right
  Conn5 : PMIOPort  Port=5  Side=Left
  Conn6 : PMIOPort  Port=6  Side=Right
  wires:
  I.M4/1 -> [IsA1]
  I.M6/1 -> [IsC1]
  V.M6/1 -> [VsC1]
  V.M5/1 -> [VsB1]
  V.M4/1 -> [VsA1]
  I.M5/1 -> [IsB1]
  I.M3/1 -> [ILC1]
  Demux2/3 -> C.I Source3/1
  Demux2/2 -> C.I Source2/1
  Demux2/1 -> C.I Source1/1
  compensation block/1(Icomp.) -> Demux2/1
  Mux4/1 -> compensation block/3(iL)
  Demux1/4 -> compensation block/2(PL)
  Mux3/1 -> compensation block/1(vL)
  Demux1/3 -> Mux3/3
  Demux1/2 -> Mux3/2
  Demux1/1 -> Mux3/1
  Demux1/7 -> Mux4/3
  Demux1/5 -> Mux4/1
  Demux1/6 -> Mux4/2
  Delay/1 -> Demux1/1
  [delay] -> Delay/2
  Mux2/1 -> Delay/1
  Demux/1 -> Mux2/2
  3-ph PQ Power/1 -> Demux/1
  Mux/1 -> Mux2/3, 3-ph PQ Power/2
  Mux1/1 -> Mux2/1, 3-ph PQ Power/1
  [VLC1] -> Mux1/3
  [VLA1] -> Mux1/1
  [VLB1] -> Mux1/2
  [ILC1] -> Mux/3
  [ILA1] -> Mux/1
  [ILB1] -> Mux/2
  V.M3/1 -> [VLC1]
  V.M2/1 -> [VLB1]
  V.M1/1 -> [VLA1]
  I.M2/1 -> [ILB1]
  I.M1/1 -> [ILA1]
  [VsB1] -> Mux6/2
  [VsA1] -> Mux6/1
  [VsC1] -> Mux6/3
  Mux6/1 -> RMS1/1, 3-ph PQ Power1/1
  RMS1/1 -> To Workspace1/1
  [IsB1] -> Mux5/2
  [IsA1] -> Mux5/1
  [IsC1] -> Mux5/3
  Mux5/1 -> RMS2/1, 3-ph PQ Power1/2
  RMS2/1 -> To Workspace2/1
  3-ph PQ Power1/1 -> Discrete  Mean value/1
  Discrete  Mean value/1 -> PF4/1(u)
  PF4/1(y) -> To Workspace3/1
  connections:
  Parallel RC1/LConn1 -- Ground9/LConn1
  Parallel RC2/LConn1 -- Ground10/LConn1
  Parallel RC3/LConn1 -- Ground11/LConn1
  Ground8/LConn1 -- V.M6/LConn2
  Ground7/LConn1 -- V.M5/LConn2
  Ground6/LConn1 -- V.M4/LConn2
  Conn5/RConn1 -- I.M6/LConn1 -- V.M6/LConn1
  Conn3/RConn1 -- I.M5/LConn1 -- V.M5/LConn1
  I.M4/LConn1 -- V.M4/LConn1 -- Conn1/RConn1
  Conn6/RConn1 -- I.M3/RConn1
  Ground3/LConn1 -- C.I Source1/LConn1
  Ground4/LConn1 -- C.I Source2/LConn1
  Ground5/LConn1 -- C.I Source3/LConn1
  Ground2/LConn1 -- V.M3/LConn2
  Ground1/LConn1 -- V.M2/LConn2
  Ground/LConn1 -- V.M1/LConn2
  Parallel RC3/RConn1 -- V.M3/LConn1 -- I.M3/LConn1 -- C.I Source3/RConn1 -- I.M6/RConn1
  Conn4/RConn1 -- I.M2/RConn1
  Parallel RC2/RConn1 -- V.M2/LConn1 -- I.M2/LConn1 -- C.I Source2/RConn1 -- I.M5/RConn1
  Conn2/RConn1 -- I.M1/RConn1
  V.M1/LConn1 -- I.M1/LConn1 -- Parallel RC1/RConn1 -- I.M4/RConn1 -- C.I Source1/RConn1

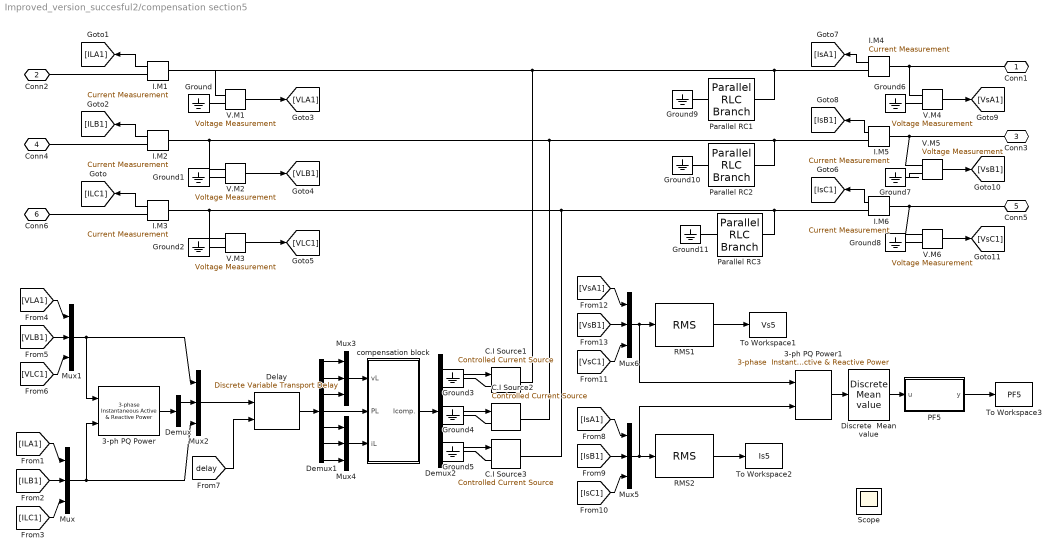
== system Improved_version_succesful2/compensation section5 ==
  3-ph PQ Power : powerlib_extras/Measurements/3-phase  Instantaneous  Active & Reactive Power  DialogController=POWERSYS.PowerSysDialog  SystemSampleTime=-1
  3-ph PQ Power1 : powerlib_extras/Measurements/3-phase  Instantaneous  Active & Reactive Power  DialogController=POWERSYS.PowerSysDialog  SystemSampleTime=-1
  C.I Source1 : powerlib/Electrical Sources/Controlled Current Source  DialogController=POWERSYS.PowerSysDialog  SystemSampleTime=-1  Initialize=on  Source_Type=AC  Amplitude=0  Phase=0  Frequency=0  Measurements=None
  C.I Source2 : powerlib/Electrical Sources/Controlled Current Source  DialogController=POWERSYS.PowerSysDialog  SystemSampleTime=-1  Initialize=on  Source_Type=AC  Amplitude=0  Phase=0  Frequency=0  Measurements=None
  C.I Source3 : powerlib/Electrical Sources/Controlled Current Source  DialogController=POWERSYS.PowerSysDialog  SystemSampleTime=-1  Initialize=on  Source_Type=AC  Amplitude=0  Phase=0  Frequency=0  Measurements=None
  Delay : powerlib_extras/Discrete  Control Blocks/Discrete Variable Transport Delay  DialogController=POWERSYS.PowerSysDialog  SystemSampleTime=-1  MaxDelay=1/40  InitialValue=0  Ts=50e-6
  Demux : Demux  Outputs=2
  Demux1 : Demux  Outputs=7
  Demux2 : Demux  Outputs=3
  Discrete  Mean value : powerlib_extras/Discrete Measurements/Discrete  Mean value  DialogController=POWERSYS.PowerSysDialog  SystemSampleTime=-1  Freq=50  Vinit=0  Ts=50e-6
  Ground{,1..11} (12 alike) : powerlib/Elements/Ground  DialogController=POWERSYS.PowerSysDialog  PhysicalDomain=powersysdomain  SubClassName=unknown  LeftPortType=p1  RightPortType=p1  LConnTagsString=a
  I.M{1..6} (6 alike) : powerlib/Measurements/Current Measurement  DialogController=POWERSYS.PowerSysDialog  SystemSampleTime=-1  PhasorSimulation=off  OutputType=Complex  PSBequivalent=0
  Mux{,1..6} (7 alike) : Mux  Inputs=3
  PF5 : Stateflow chart
  Parallel RC1 : powerlib/Elements/Parallel RLC Branch  DialogController=POWERSYS.PowerSysDialog  PhysicalDomain=powersysdomain  SubClassName=unknown  LeftPortType=p1  RightPortType=p1  LConnTagsString=a  RConnTagsString=__new0  BranchType=RC  Resistance=100  Inductance=1e-3  SetiL0=off  InitialCurrent=0  Capacitance=1/(10000*pi)  Setx0=off  InitialVoltage=0  Measurements=None
  Parallel RC2 : powerlib/Elements/Parallel RLC Branch  DialogController=POWERSYS.PowerSysDialog  PhysicalDomain=powersysdomain  SubClassName=unknown  LeftPortType=p1  RightPortType=p1  LConnTagsString=a  RConnTagsString=__new0  BranchType=RC  Resistance=100  Inductance=1e-3  SetiL0=off  InitialCurrent=0  Capacitance=1/(10000*pi)  Setx0=off  InitialVoltage=0  Measurements=None
  Parallel RC3 : powerlib/Elements/Parallel RLC Branch  DialogController=POWERSYS.PowerSysDialog  PhysicalDomain=powersysdomain  SubClassName=unknown  LeftPortType=p1  RightPortType=p1  LConnTagsString=a  RConnTagsString=__new0  BranchType=RC  Resistance=100  Inductance=1e-3  SetiL0=off  InitialCurrent=0  Capacitance=1/(10000*pi)  Setx0=off  InitialVoltage=0  Measurements=None
  RMS1 : powerlib_extras/Measurements/RMS  DialogController=POWERSYS.PowerSysDialog  SystemSampleTime=-1  f1=50
  RMS2 : powerlib_extras/Measurements/RMS  DialogController=POWERSYS.PowerSysDialog  SystemSampleTime=-1  f1=50
  Scope : Scope
      settings: YMin=2  YMax=6
  To Workspace1 : ToWorkspace  VariableName=Vs5  SampleTime=y  SaveFormat=Array
  To Workspace2 : ToWorkspace  VariableName=Is5  SampleTime=y  SaveFormat=Array
  To Workspace3 : ToWorkspace  VariableName=PF5  SampleTime=y  SaveFormat=Array
  V.M{1..6} (6 alike) : powerlib/Measurements/Voltage Measurement  DialogController=POWERSYS.PowerSysDialog  SystemSampleTime=-1  PhasorSimulation=off  OutputType=Complex  PSBequivalent=0
  compensation block : Subsystem
  Conn1 : PMIOPort  Port=1  Side=Left
  Conn2 : PMIOPort  Port=2  Side=Right
  Conn3 : PMIOPort  Port=3  Side=Left
  Conn4 : PMIOPort  Port=4  Side=Right
  Conn5 : PMIOPort  Port=5  Side=Left
  Conn6 : PMIOPort  Port=6  Side=Right
  wires:
  I.M1/1 -> [ILA1]
  I.M2/1 -> [ILB1]
  V.M1/1 -> [VLA1]
  V.M2/1 -> [VLB1]
  V.M3/1 -> [VLC1]
  [ILB1] -> Mux/2
  [ILA1] -> Mux/1
  [ILC1] -> Mux/3
  [VLB1] -> Mux1/2
  [VLA1] -> Mux1/1
  [VLC1] -> Mux1/3
  Mux1/1 -> 3-ph PQ Power/1, Mux2/1
  Mux/1 -> 3-ph PQ Power/2, Mux2/3
  3-ph PQ Power/1 -> Demux/1
  Demux/1 -> Mux2/2
  Mux2/1 -> Delay/1
  [delay] -> Delay/2
  Delay/1 -> Demux1/1
  Demux1/6 -> Mux4/2
  Demux1/5 -> Mux4/1
  Demux1/7 -> Mux4/3
  Demux1/1 -> Mux3/1
  Demux1/2 -> Mux3/2
  Demux1/3 -> Mux3/3
  Mux3/1 -> compensation block/1(vL)
  Demux1/4 -> compensation block/2(PL)
  Mux4/1 -> compensation block/3(iL)
  compensation block/1(Icomp.) -> Demux2/1
  Demux2/1 -> C.I Source1/1
  Demux2/2 -> C.I Source2/1
  Demux2/3 -> C.I Source3/1
  I.M3/1 -> [ILC1]
  I.M5/1 -> [IsB1]
  V.M4/1 -> [VsA1]
  V.M5/1 -> [VsB1]
  V.M6/1 -> [VsC1]
  I.M6/1 -> [IsC1]
  I.M4/1 -> [IsA1]
  [VsB1] -> Mux6/2
  [VsA1] -> Mux6/1
  [VsC1] -> Mux6/3
  Mux6/1 -> RMS1/1, 3-ph PQ Power1/1
  RMS1/1 -> To Workspace1/1
  [IsB1] -> Mux5/2
  [IsA1] -> Mux5/1
  [IsC1] -> Mux5/3
  Mux5/1 -> RMS2/1, 3-ph PQ Power1/2
  RMS2/1 -> To Workspace2/1
  3-ph PQ Power1/1 -> Discrete  Mean value/1
  Discrete  Mean value/1 -> PF5/1(u)
  PF5/1(y) -> To Workspace3/1
  connections:
  I.M1/LConn1 -- V.M1/LConn1 -- I.M4/RConn1 -- Parallel RC1/RConn1 -- C.I Source1/RConn1
  Conn2/RConn1 -- I.M1/RConn1
  I.M5/RConn1 -- C.I Source2/RConn1 -- I.M2/LConn1 -- V.M2/LConn1 -- Parallel RC2/RConn1
  Conn4/RConn1 -- I.M2/RConn1
  I.M6/RConn1 -- C.I Source3/RConn1 -- I.M3/LConn1 -- V.M3/LConn1 -- Parallel RC3/RConn1
  Ground/LConn1 -- V.M1/LConn2
  Ground1/LConn1 -- V.M2/LConn2
  Ground2/LConn1 -- V.M3/LConn2
  Ground5/LConn1 -- C.I Source3/LConn1
  Ground4/LConn1 -- C.I Source2/LConn1
  Ground3/LConn1 -- C.I Source1/LConn1
  Conn6/RConn1 -- I.M3/RConn1
  Conn1/RConn1 -- V.M4/LConn1 -- I.M4/LConn1
  V.M5/LConn1 -- I.M5/LConn1 -- Conn3/RConn1
  V.M6/LConn1 -- I.M6/LConn1 -- Conn5/RConn1
  Ground6/LConn1 -- V.M4/LConn2
  Ground7/LConn1 -- V.M5/LConn2
  Ground8/LConn1 -- V.M6/LConn2
  Parallel RC3/LConn1 -- Ground11/LConn1
  Parallel RC2/LConn1 -- Ground10/LConn1
  Parallel RC1/LConn1 -- Ground9/LConn1

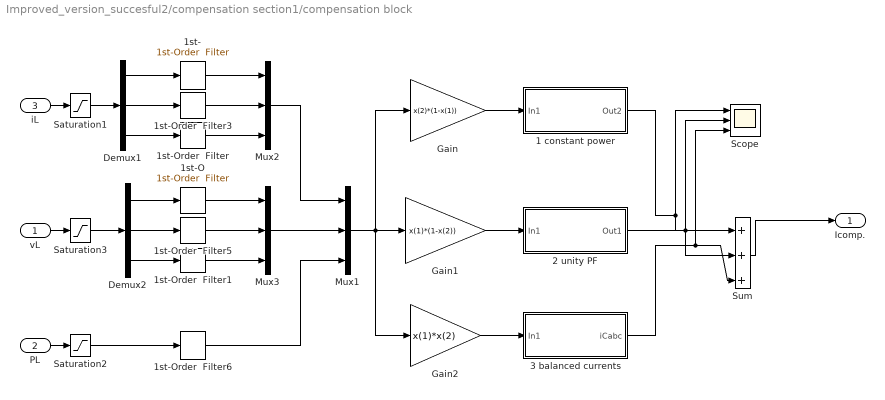
== system Improved_version_succesful2/compensation section1/compensation block ==
  vL : Inport  OutDataType=fixdt(1, 16)  OutScaling=2^0
  PL : Inport  Port=2  OutDataType=fixdt(1, 16)  OutScaling=2^0
  iL : Inport  Port=3  OutDataType=fixdt(1, 16)  OutScaling=2^0
  1 constant power : Subsystem
  1st- : powerlib_extras/Control  Blocks/1st-Order  Filter  DialogController=POWERSYS.PowerSysDialog  SystemSampleTime=-1  FilterType=Lowpass  Tc=.00051  Initialize=off  Vac_Init=[0.8 -25 60]  Vdc_Init=-0.4  PlotResponse=off  param1=[1 500 1]
  1st-O : powerlib_extras/Control  Blocks/1st-Order  Filter  DialogController=POWERSYS.PowerSysDialog  SystemSampleTime=-1  FilterType=Lowpass  Tc=.00051  Initialize=off  Vac_Init=[0.8 -25 60]  Vdc_Init=-0.4  PlotResponse=off  param1=[1 500 1]
  1st-Order  Filter{,1,3,5..6} (5 alike) : powerlib_extras/Control  Blocks/1st-Order  Filter  DialogController=POWERSYS.PowerSysDialog  SystemSampleTime=-1  FilterType=Lowpass  Tc=.00051  Initialize=off  Vac_Init=[0.8 -25 60]  Vdc_Init=-0.4  PlotResponse=off  param1=[1 500 1]
  2 unity PF : Subsystem
  "3 balanced currents " : Subsystem
  Demux1 : Demux  Outputs=3
  Demux2 : Demux  Outputs=3
  Gain : Gain  Gain=x(2)*(1-x(1))  ParameterDataType=fixdt(1, 16)  ParameterScaling=2^0  OutDataType=fixdt(1, 16)  OutScaling=2^0
  Gain1 : Gain  Gain=x(1)*(1-x(2))  ParameterDataType=fixdt(1, 16)  ParameterScaling=2^0  OutDataType=fixdt(1, 16)  OutScaling=2^0
  Gain2 : Gain  Gain=x(1)*x(2)  ParameterDataType=fixdt(1, 16)  ParameterScaling=2^0  OutDataType=fixdt(1, 16)  OutScaling=2^0
  Mux1 : Mux  Inputs=3
  Mux2 : Mux  Inputs=3
  Mux3 : Mux  Inputs=3
  Saturation1 : Saturate  UpperLimit=100  LowerLimit=-100  OutDataType=sfix(16)  OutScaling=2^0
  Saturation2 : Saturate  UpperLimit=10000  LowerLimit=0  OutDataType=sfix(16)  OutScaling=2^0
  Saturation3 : Saturate  UpperLimit=500  LowerLimit=-500  OutDataType=sfix(16)  OutScaling=2^0
  Scope : Scope  NumInputPorts=3
      settings: YMin=-7.5~-1~-1  YMax=10~1~1  SaveName=ScopeData33
  Sum : Sum  Inputs=|+++  OutDataType=fixdt(1, 16)  OutScaling=2^0
  Icomp. : Outport  OutDataType=sfix(16)  OutScaling=2^0
  wires:
  vL/1 -> Saturation3/1
  Demux1/1 -> 1st-/1
  Demux1/2 -> 1st-Order  Filter3/1
  Demux1/3 -> 1st-Order  Filter/1
  Saturation1/1 -> Demux1/1
  1st-Order  Filter1/1 -> Mux3/3
  Demux2/1 -> 1st-O/1
  Demux2/2 -> 1st-Order  Filter5/1
  Demux2/3 -> 1st-Order  Filter1/1
  1st-O/1 -> Mux3/1
  1st-Order  Filter5/1 -> Mux3/2
  Saturation2/1 -> 1st-Order  Filter6/1
  1st-/1 -> Mux2/1
  1st-Order  Filter3/1 -> Mux2/2
  1st-Order  Filter/1 -> Mux2/3
  Saturation3/1 -> Demux2/1
  iL/1 -> Saturation1/1
  PL/1 -> Saturation2/1
  Mux3/1 -> Mux1/2
  Mux2/1 -> Mux1/1
  1st-Order  Filter6/1 -> Mux1/3
  Gain/1 -> 1 constant power/1(In1)
  Mux1/1 -> Gain/1, Gain1/1, Gain2/1
  Gain1/1 -> 2 unity PF/1(In1)
  1 constant power/1(Out2) -> Sum/1, Scope/1
  2 unity PF/1(Out1) -> Sum/2, Scope/2
  Gain2/1 -> "3 balanced currents "/1(In1)
  "3 balanced currents "/1(iCabc) -> Sum/3, Scope/3
  Sum/1 -> Icomp./1

== system Improved_version_succesful2/compensation section2/compensation block ==
  vL : Inport  OutDataType=fixdt(1, 16)  OutScaling=2^0
  PL : Inport  Port=2  OutDataType=fixdt(1, 16)  OutScaling=2^0
  iL : Inport  Port=3  OutDataType=fixdt(1, 16)  OutScaling=2^0
  1 constant power : Subsystem
  1st- : powerlib_extras/Control  Blocks/1st-Order  Filter  DialogController=POWERSYS.PowerSysDialog  SystemSampleTime=-1  FilterType=Lowpass  Tc=.00051  Initialize=off  Vac_Init=[0.8 -25 60]  Vdc_Init=-0.4  PlotResponse=off  param1=[1 500 1]
  1st-O : powerlib_extras/Control  Blocks/1st-Order  Filter  DialogController=POWERSYS.PowerSysDialog  SystemSampleTime=-1  FilterType=Lowpass  Tc=.00051  Initialize=off  Vac_Init=[0.8 -25 60]  Vdc_Init=-0.4  PlotResponse=off  param1=[1 500 1]
  1st-Order  Filter{,1,3,5..6} (5 alike) : powerlib_extras/Control  Blocks/1st-Order  Filter  DialogController=POWERSYS.PowerSysDialog  SystemSampleTime=-1  FilterType=Lowpass  Tc=.00051  Initialize=off  Vac_Init=[0.8 -25 60]  Vdc_Init=-0.4  PlotResponse=off  param1=[1 500 1]
  2 unity PF : Subsystem
  "3 balanced currents " : Subsystem
  Demux1 : Demux  Outputs=3
  Demux2 : Demux  Outputs=3
  Gain : Gain  Gain=x(4)*(1-x(3))  ParameterDataType=fixdt(1, 16)  ParameterScaling=2^0  OutDataType=fixdt(1, 16)  OutScaling=2^0
  Gain1 : Gain  Gain=x(3)*(1-x(4))  ParameterDataType=fixdt(1, 16)  ParameterScaling=2^0  OutDataType=fixdt(1, 16)  OutScaling=2^0
  Gain2 : Gain  Gain=x(3)*x(4)  ParameterDataType=fixdt(1, 16)  ParameterScaling=2^0  OutDataType=fixdt(1, 16)  OutScaling=2^0
  Mux1 : Mux  Inputs=3
  Mux2 : Mux  Inputs=3
  Mux3 : Mux  Inputs=3
  Saturation1 : Saturate  UpperLimit=100  LowerLimit=-100  OutDataType=sfix(16)  OutScaling=2^0
  Saturation2 : Saturate  UpperLimit=10000  LowerLimit=0  OutDataType=sfix(16)  OutScaling=2^0
  Saturation3 : Saturate  UpperLimit=500  LowerLimit=-500  OutDataType=sfix(16)  OutScaling=2^0
  Scope : Scope  NumInputPorts=3
      settings: YMin=-7.5~-1~-1  YMax=10~1~1  SaveName=ScopeData33
  Sum : Sum  Inputs=|+++  OutDataType=fixdt(1, 16)  OutScaling=2^0
  Icomp. : Outport  OutDataType=sfix(16)  OutScaling=2^0
  wires:
  Sum/1 -> Icomp./1
  "3 balanced currents "/1(iCabc) -> Scope/3, Sum/3
  Gain2/1 -> "3 balanced currents "/1(In1)
  2 unity PF/1(Out1) -> Scope/2, Sum/2
  1 constant power/1(Out2) -> Scope/1, Sum/1
  Gain1/1 -> 2 unity PF/1(In1)
  Mux1/1 -> Gain2/1, Gain1/1, Gain/1
  Gain/1 -> 1 constant power/1(In1)
  1st-Order  Filter6/1 -> Mux1/3
  Mux2/1 -> Mux1/1
  Mux3/1 -> Mux1/2
  PL/1 -> Saturation2/1
  iL/1 -> Saturation1/1
  Saturation3/1 -> Demux2/1
  1st-Order  Filter/1 -> Mux2/3
  1st-Order  Filter3/1 -> Mux2/2
  1st-/1 -> Mux2/1
  Saturation2/1 -> 1st-Order  Filter6/1
  1st-Order  Filter5/1 -> Mux3/2
  1st-O/1 -> Mux3/1
  Demux2/3 -> 1st-Order  Filter1/1
  Demux2/2 -> 1st-Order  Filter5/1
  Demux2/1 -> 1st-O/1
  1st-Order  Filter1/1 -> Mux3/3
  Saturation1/1 -> Demux1/1
  Demux1/3 -> 1st-Order  Filter/1
  Demux1/2 -> 1st-Order  Filter3/1
  Demux1/1 -> 1st-/1
  vL/1 -> Saturation3/1
